simulink model "still_to_implement_controlling"  (R2024b)
settings: Solver=FixedStepAuto  StartTime=0.0  StopTime=inf  FixedStep=0.01  RelTol=1e-3  EnableMultiTasking=on
InitFcn:
  | breakp=[-1, -0.9, -0.8, -0.6, -0.4, -0.2, -0.1, 0, 0.1, 0.2, 0.4, 0.6, 0.8, 1];
  | 
  | splinenew =[-1, -0.92, -0.8, -0.50, -0.28, -0.12, -0.05, 0, 0.005, 0.01, 0.02, 0.025,0.03,0.035];
model workspace (MAT data in the model file):
  threshDetectGP = 0.1
libraries: simulink x22, arduinolib x6, dspswit3 x5, arduinosensorlib x2
(part 2 of 2)

== system still_to_implement_controlling/Subsystem3/Right Motor Velocity/Subsystem/CAN Pack1/Subsystem/Buff 5 ==
  In2 : Inport
  Constant2 : Constant  Value=4  OutDataTypeStr=uint16
  Data Type Conversion5 : DataTypeConversion  OutDataTypeStr=uint8  SaturateOnIntegerOverflow=off  RndMeth=Floor
  Shift Arithmetic5 : ArithShift  BitShiftNumberSource=Input port  BitShiftNumber=8  BitShiftDirection=Right
      settings: InputPortMap=u0,p1
  Out1 : Outport
  wires:
  In2/1 -> Shift Arithmetic5/1
  Shift Arithmetic5/1 -> Data Type Conversion5/1
  Data Type Conversion5/1 -> Out1/1
  Constant2/1 -> Shift Arithmetic5/2

== system still_to_implement_controlling/Subsystem3/Right Motor Velocity/Subsystem/CAN Pack1/Subsystem/Buff 6 ==
  In3 : Inport
  In4 : Inport  Port=2
  Bitwise AND2 : simulink/Logic and Bit Operations/Bitwise Operator  logicop=AND  UseBitMask=on  BitMask=bin2dec('000000001111')  BitMaskRealWorld=Stored Integer
  Bitwise OR2 : simulink/Logic and Bit Operations/Bitwise Operator  logicop=OR  UseBitMask=off  NumInputPorts=2  BitMask=bin2dec('11011001')  BitMaskRealWorld=Stored Integer
  Constant1 : Constant  Value=8  OutDataTypeStr=uint16
  Constant2 : Constant  Value=4  OutDataTypeStr=uint16
  Data Type Conversion6 : DataTypeConversion  OutDataTypeStr=uint8  SaturateOnIntegerOverflow=off  RndMeth=Floor
  Shift Arithmetic6 : ArithShift  BitShiftNumberSource=Input port  BitShiftNumber=8  BitShiftDirection=Left
      settings: InputPortMap=u0,p1
  Shift Arithmetic7 : ArithShift  BitShiftNumberSource=Input port  BitShiftNumber=8  BitShiftDirection=Right
      settings: InputPortMap=u0,p1
  Out1 : Outport
  wires:
  In4/1 -> Shift Arithmetic7/1
  Shift Arithmetic7/1 -> Bitwise OR2/2
  Shift Arithmetic6/1 -> Bitwise OR2/1
  Bitwise OR2/1 -> Data Type Conversion6/1
  In3/1 -> Bitwise AND2/1
  Bitwise AND2/1 -> Shift Arithmetic6/1
  Data Type Conversion6/1 -> Out1/1
  Constant2/1 -> Shift Arithmetic6/2
  Constant1/1 -> Shift Arithmetic7/2

== system still_to_implement_controlling/Subsystem3/Right Motor Velocity/Subsystem/CAN Pack1/Subsystem/Buff 7 ==
  In1 : Inport
  Bitwise AND4 : simulink/Logic and Bit Operations/Bitwise Operator  logicop=AND  UseBitMask=on  BitMask=bin2dec('000011111111')  BitMaskRealWorld=Stored Integer
  Data Type Conversion7 : DataTypeConversion  OutDataTypeStr=uint8  SaturateOnIntegerOverflow=off  RndMeth=Floor
  Out1 : Outport
  wires:
  Bitwise AND4/1 -> Data Type Conversion7/1
  Data Type Conversion7/1 -> Out1/1
  In1/1 -> Bitwise AND4/1

== stateflow chart still_to_implement_controlling/Subsystem3/Chart ==
  state Reset
    vel = 0;
    enablestati=0;
  state Tensioning
    enablestati = 1;
    vel = -3;
  state Stop
    vel = 0;
  state Disable
    enablestati = -1;
  (default) -> Reset
  Reset -> Tensioning : [ON_OFF == 1]
  Tensioning -> Disable [order 2] : [ON_OFF == 0]
  Tensioning -> Stop [order 1] : [MOTOR_TORQUE >= 0.85]
  Stop -> Disable : after(1,sec)
  data: MOTOR_TORQUE input; ON_OFF input; thrtorque local; enablestati output; vel output

== stateflow chart still_to_implement_controlling/Subsystem3/Chart1 ==
  state Reset
    vel = 0;
    enablestati=0;
  state Tensioning
    enablestati = 1;
    vel = 3;
  state Stop
    vel = 0;
  state Disable
    enablestati = -1;
  (default) -> Reset
  Reset -> Tensioning : [ON_OFF == 1]
  Tensioning -> Disable [order 2] : [ON_OFF == 0]
  Tensioning -> Stop [order 1] : [MOTOR_TORQUE >= 0.85]
  Stop -> Disable : after(1,sec)
  data: MOTOR_TORQUE input; ON_OFF input; thrtorque local; enablestati output; vel output
